simulink model "Day_07_LQR_with_Energy_Shaping"  (R2024a)
settings: Solver=daessc  StartTime=0.0  StopTime=5  RelTol=1e-3
values from neighbouring files (symbols this model uses):
  D0 = 2700    [Day_07.m]
  D1 = 2700    [Day_07.m]
  K = 20    [Day_07.m]
  K_LQR = lqr(A, B, Q, R)    [Day_07.m]
  L0 = 0.01    [Day_07.m]
  L1 = 0.14    [Day_07.m]
  limit = 0.45    [Day_07.m]
  M1 = L1*W1*T1*D1    (= 0.0378)    [Day_07.m]
  T0 = 0.01    [Day_07.m]
  T1 = 0.01    [Day_07.m]
  W0 = 0.01    [Day_07.m]
  W1 = 0.01    [Day_07.m]
  x1_d = 0    [Day_07.m]
  x2_d = 0    [Day_07.m]
  x3_d = 0    [Day_07.m]
  x4_d = 0    [Day_07.m]
undefined symbols (not defined in the file or in its folder): X, Y, Z
libraries: sm_lib x14, nesl_utility x7
settings Model: Creator=mingeun  LastModifiedBy=mingeun
settings DataIOCC: ReturnWorkspaceOutputs=off
settings OptimizationCC: BlockReduction=off  DefaultParameterBehavior=Inlined  BufferReuse=off

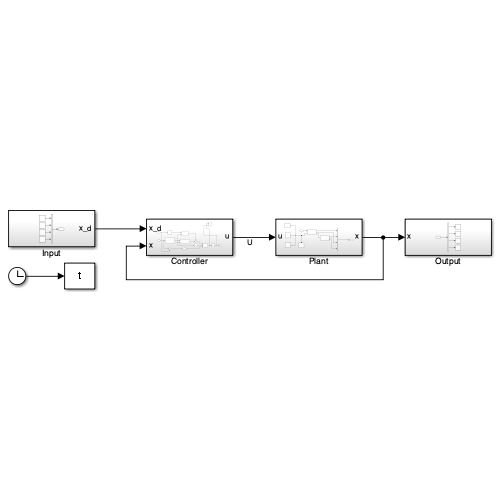
[thumbnail: Simulink's stored preview of the top-level diagram]
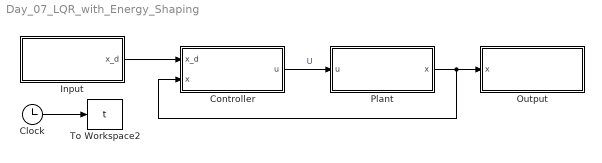
== system Day_07_LQR_with_Energy_Shaping ==
  Clock : Clock
  Controller : Subsystem
  Input : Subsystem
  Output : Subsystem
  Plant : Subsystem
  To Workspace2 : ToWorkspace  VariableName=t  SampleTime=-1
  wires:
  Clock/1 -> To Workspace2/1
  Input/1(x_d) -> Controller/1(x_d)
  Controller/1(u) -> Plant/1(u)  "U"
  Plant/1(x) -> Output/1(x), Controller/2(x)

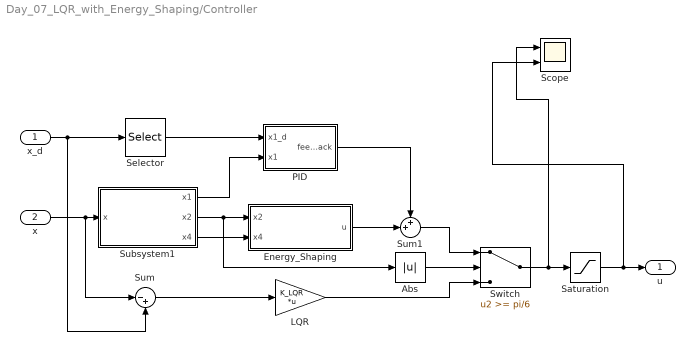
== system Day_07_LQR_with_Energy_Shaping/Controller ==
  x_d : Inport
  x : Inport  Port=2
  Abs : Abs  SaturateOnIntegerOverflow=off
  Energy_Shaping : Subsystem
  LQR : Gain  Gain=K_LQR  Multiplication=Matrix(K*u)
  PID : Subsystem  mask{Kp=2, Ki=0.02, Kd=0.2}
  Saturation : Saturate  UpperLimit=limit  LowerLimit=-limit
  Scope : Scope  NumInputPorts=2
  Selector : Selector  InputPortWidth=4  IndexOptions=Index vector (dialog)  Indices=1  OutputSizes=1
  Subsystem1 : Subsystem
  Sum : Sum  Inputs=|-+
  Sum1 : Sum  Inputs=++|
  Switch : Switch  Threshold=pi/6  SaturateOnIntegerOverflow=off  InputSameDT=off
  u : Outport
  wires:
  Switch/1 -> Scope/1, Saturation/1
  x_d/1 -> Sum/2, Selector/1
  Abs/1 -> Switch/2
  Sum1/1 -> Switch/1
  x/1 -> Subsystem1/1(x), Sum/1
  Subsystem1/3(x4) -> Energy_Shaping/2(x4)
  Energy_Shaping/1(u) -> Sum1/2
  Subsystem1/2(x2) -> Energy_Shaping/1(x2), Abs/1
  Subsystem1/1(x1) -> PID/2(x1)
  Sum/1 -> LQR/1
  Selector/1 -> PID/1(x1_d)
  PID/1(feedback) -> Sum1/1
  LQR/1 -> Switch/3
  Saturation/1 -> Scope/2, u/1

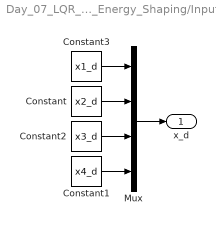
== system Day_07_LQR_with_Energy_Shaping/Input ==
  Constant : Constant  Value=x2_d
  Constant1 : Constant  Value=x4_d
  Constant2 : Constant  Value=x3_d
  Constant3 : Constant  Value=x1_d
  Mux : Mux
  x_d : Outport
  wires:
  Mux/1 -> x_d/1
  Constant1/1 -> Mux/4
  Constant2/1 -> Mux/3
  Constant/1 -> Mux/2
  Constant3/1 -> Mux/1

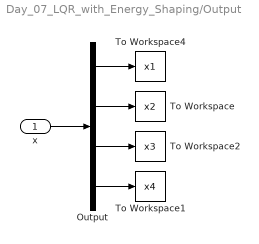
== system Day_07_LQR_with_Energy_Shaping/Output ==
  x : Inport
  Output : Demux
  To Workspace : ToWorkspace  VariableName=x2  SampleTime=-1
  To Workspace1 : ToWorkspace  VariableName=x4  SampleTime=-1
  To Workspace2 : ToWorkspace  VariableName=x3  SampleTime=-1
  To Workspace4 : ToWorkspace  VariableName=x1  SampleTime=-1
  wires:
  Output/3 -> To Workspace2/1
  Output/4 -> To Workspace1/1
  Output/2 -> To Workspace/1
  Output/1 -> To Workspace4/1
  x/1 -> Output/1

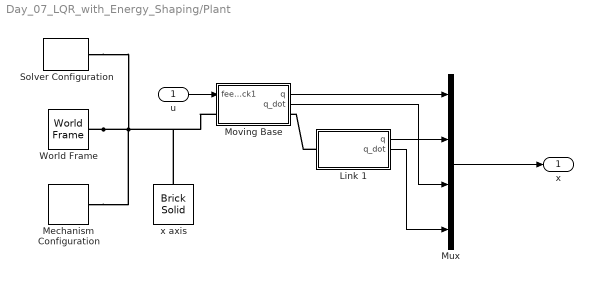
== system Day_07_LQR_with_Energy_Shaping/Plant ==
  u : Inport
  Link 1 : Subsystem  mask{L=L1*100, W=W1*100, H=T1*100, rho=D1, rgb=[0.25 0.40 0.70], angle=180, F=0.1}
      mask prompts: L "Length (cm)"; W "Width (cm)"; H "Thickness (cm)"; rho "Density (kg/m^3)"; rgb "Color [R G B]"; angle "Initial Angle (degree)"; F "Disturbance [N]"
  Mechanism Configuration : sm_lib/Utilities/Mechanism Configuration  UniformGravity=Constant  GravityVector=[0 0 -9.80665]  GravityVectorUnits=m/s^2  LinearizationDelta=0.001  JointModeTransitionNonlinearIterations=2
  Moving Base : Subsystem  mask{L=L0*100, W=W0*100, H=T0*100, rho=D0, RGB=[0.8 0.45 0.0]}
      mask prompts: L "Length (cm)"; W "Width (cm)"; H "Thickness (cm)"; rho "Density (kg/m^3)"; RGB "Color [R G B]"
  Mux : Mux
  Solver Configuration : nesl_utility/Solver Configuration  PhysicalDomain=network_engine_domain  SubClassName=solver  LeftPortType=input  RightPortType=generic  Tones=[]  Harmonics=[]  SimulateNoise=off  Profile=off  UseLocalSampling=off  EnableSwitchedLinearOptims=on  FrequencyDomain=off  UseCCode=off  RelTol=0.001  AbsTol=0.001  MinStep=1e-09  ToWorkspace=off  RevertToSquareIcSolve=off  NumHomotopyIterations=100  PhasorMode=off  PhasorModeNumHarmonics=1  ConsistencySolver=NEWTON_XTOL_AFTER_FTOL  IndexReductionMethod=DerivativeReplacement  DoDC=off  ResidualTolerance=1e-09  ConsistencyTolSource=GLOBAL  ConsistencyAbsTol=0.001  ConsistencyRelTol=0.001  ConsistencyTolFactor=0.001  UseLocalSolver=off  LocalSolverChoice=NE_BACKWARD_EULER_ADVANCER  ResolveIndetEquations=on  FunctionEvalNumThread=1  LocalSolverSampleTime=0.001  DoFixedCost=off  MaxNonlinIter=3  MaxModeIter=2  ComputeImpulses=off  ImpulseIterations=2  LinearAlgebra=auto  LinearAlgebraNumThread=0  EquationFormulation=NE_TIME_EF  DelaysMemoryBudget=1024  AutomaticFiltering=on  FilteringTimeConstant=0.001  PartitionStorageMethod=AS_NEEDED  PartitionMemoryBudget=1024  PartitionMethod=ROBUST  MultibodyUseLocalSolver=off  MultibodyLocalSolverChoice=ODE1  MultibodyLocalSolverSampleTime=0.001
  World Frame : sm_lib/Frames and Transforms/World Frame
  x axis : sm_lib/Body Elements/Brick Solid  BrickDimensions=[1000 1 1]  BrickDimensionsUnits=mm  ExportEntireGeometry=off  InertiaType=CalculateFromGeometry  BasedOnType=Density  Density=1000  DensityUnits=kg/m^3  Mass=1  MassUnits=kg  CenterOfMass=[0 0 0]  CenterOfMassUnits=m  MomentsOfInertia=[1 1 1]  MomentsOfInertiaUnits=kg*m^2  ProductsOfInertia=[0 0 0]  ProductsOfInertiaUnits=kg*m^2  GraphicType=FromGeometry  MarkerShape=Sphere  MarkerSize=10  GraphicVisPropType=SimpleVisualProperties  GraphicDiffuseColor=[0.0 0.0 0.0]  GraphicOpacity=1  GraphicSpecularColor=[0.5 0.5 0.5 1.0]  GraphicAmbientColor=[0.15 0.15 0.15 1.0]  GraphicEmissiveColor=[0.0 0.0 0.0 1.0]  GraphicShininess=75  DoExposeReferenceFrame=on  SerializedFrames=<Frames/>
  x : Outport
  wires:
  Moving Base/1(q) -> Mux/1
  Link 1/1(q) -> Mux/2
  u/1 -> Moving Base/1(feedback1)
  Link 1/2(q_dot) -> Mux/4
  Moving Base/2(q_dot) -> Mux/3
  Mux/1 -> x/1
  connections:
  World Frame/RConn1 -- Solver Configuration/RConn1 -- Moving Base/LConn1 -- x axis/RConn1 -- Mechanism Configuration/RConn1
  Link 1/LConn1 -- Moving Base/RConn1

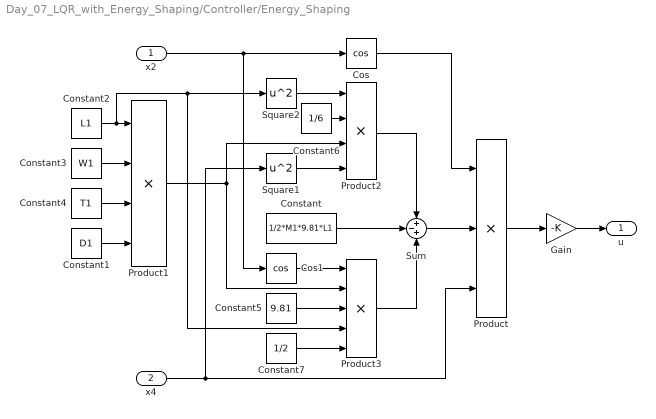
== system Day_07_LQR_with_Energy_Shaping/Controller/Energy_Shaping ==
  x2 : Inport
  x4 : Inport  Port=2
  Constant : Constant  Value=1/2*M1*9.81*L1
  Constant1 : Constant  Value=D1
  Constant2 : Constant  Value=L1
  Constant3 : Constant  Value=W1
  Constant4 : Constant  Value=T1
  Constant5 : Constant  Value=9.81
  Constant6 : Constant  Value=1/6
  Constant7 : Constant  Value=1/2
  Cos : Trigonometry  Operator=cos
  Cos1 : Trigonometry  Operator=cos
  Gain : Gain  Gain=-K
  Product : Product  Inputs=3
  Product1 : Product  Inputs=4
  Product2 : Product  Inputs=4
  Product3 : Product  Inputs=5
  Square1 : Math  Operator=square  SignedPower=on  RndMeth=Zero
  Square2 : Math  Operator=square  SignedPower=on  RndMeth=Zero
  Sum : Sum  Inputs=+-+
  u : Outport
  wires:
  Gain/1 -> u/1
  Sum/1 -> Product/2
  Cos/1 -> Product/1
  Product/1 -> Gain/1
  x4/1 -> Product/3, Square1/1
  x2/1 -> Cos1/1, Cos/1
  Constant2/1 -> Product3/4, Square2/1, Product1/1
  Constant3/1 -> Product1/2
  Constant4/1 -> Product1/3
  Constant1/1 -> Product1/4
  Product1/1 -> Product3/2, Product2/3
  Square1/1 -> Product2/4
  Product2/1 -> Sum/1
  Cos1/1 -> Product3/1
  Constant7/1 -> Product3/5
  Constant5/1 -> Product3/3
  Constant6/1 -> Product2/2
  Square2/1 -> Product2/1
  Constant/1 -> Sum/2
  Product3/1 -> Sum/3

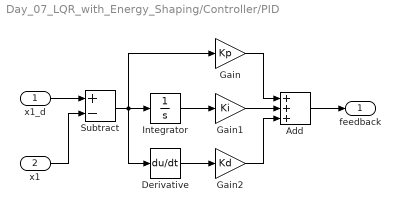
== system Day_07_LQR_with_Energy_Shaping/Controller/PID ==
  x1_d : Inport
  x1 : Inport  Port=2
  Add : Sum  Inputs=+++
  Derivative : Derivative
  Gain : Gain  Gain=Kp
  Gain1 : Gain  Gain=Ki
  Gain2 : Gain  Gain=Kd
  Integrator : Integrator
  Subtract : Sum  Inputs=+-
  feedback : Outport
  wires:
  x1_d/1 -> Subtract/1
  Derivative/1 -> Gain2/1
  Subtract/1 -> Integrator/1, Gain/1, Derivative/1
  Integrator/1 -> Gain1/1
  Add/1 -> feedback/1
  Gain/1 -> Add/1
  Gain2/1 -> Add/3
  Gain1/1 -> Add/2
  x1/1 -> Subtract/2

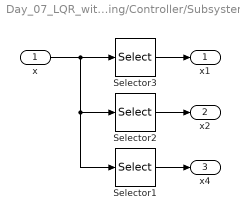
== system Day_07_LQR_with_Energy_Shaping/Controller/Subsystem1 ==
  x : Inport
  Selector1 : Selector  InputPortWidth=4  IndexOptions=Index vector (dialog)  Indices=4  OutputSizes=1
  Selector2 : Selector  InputPortWidth=4  IndexOptions=Index vector (dialog)  Indices=2  OutputSizes=1
  Selector3 : Selector  InputPortWidth=4  IndexOptions=Index vector (dialog)  Indices=1  OutputSizes=1
  x1 : Outport
  x2 : Outport  Port=2
  x4 : Outport  Port=3
  wires:
  Selector1/1 -> x4/1
  Selector2/1 -> x2/1
  Selector3/1 -> x1/1
  x/1 -> Selector2/1, Selector1/1, Selector3/1

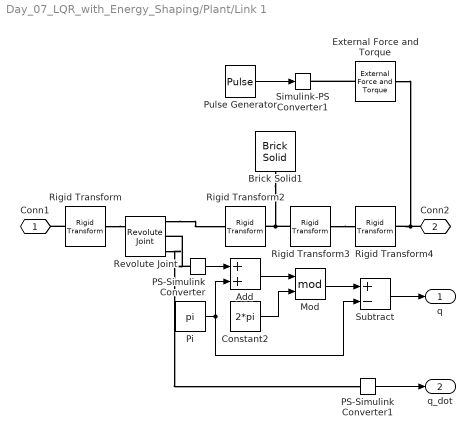
== system Day_07_LQR_with_Energy_Shaping/Plant/Link 1 ==
  Add : Sum
  Brick Solid1 : sm_lib/Body Elements/Brick Solid  BrickDimensions=[L W H]  BrickDimensionsUnits=cm  ExportEntireGeometry=off  InertiaType=CalculateFromGeometry  BasedOnType=Density  Density=rho  DensityUnits=kg/m^3  Mass=1  MassUnits=kg  CenterOfMass=[0 0 0]  CenterOfMassUnits=m  MomentsOfInertia=[1 1 1]  MomentsOfInertiaUnits=kg*m^2  ProductsOfInertia=[0 0 0]  ProductsOfInertiaUnits=kg*m^2  GraphicType=FromGeometry  MarkerShape=Sphere  MarkerSize=10  GraphicVisPropType=SimpleVisualProperties  GraphicDiffuseColor=rgb  GraphicOpacity=1  GraphicSpecularColor=[0.5 0.5 0.5 1.0]  GraphicAmbientColor=[0.15 0.15 0.15 1.0]  GraphicEmissiveColor=[0.0 0.0 0.0 1.0]  GraphicShininess=75  DoExposeReferenceFrame=on  SerializedFrames=<Frames/>
  Constant2 : Constant  Value=2*pi
  External Force and Torque : sm_lib/Forces and Torques/External Force and Torque  EnableForceX=on  EnableForceY=off  EnableForceZ=off  EnableForce=off  ForceResolutionFrame=World  EnableTorqueX=off  EnableTorqueY=off  EnableTorqueZ=off  EnableTorque=off  TorqueResolutionFrame=World
  Mod : Math  Operator=mod  OutputSignalType=real
  PS-Simulink Converter : nesl_utility/PS-Simulink Converter  PhysicalDomain=network_engine_domain  SubClassName=ps_output  LeftPortType=input  RightPortType=output  PseudoPeriodic=off  Frequencies=[]  VectorFormat=inherit  Unit=inherit  AffineConversion=off
  PS-Simulink Converter1 : nesl_utility/PS-Simulink Converter  PhysicalDomain=network_engine_domain  SubClassName=ps_output  LeftPortType=input  RightPortType=output  PseudoPeriodic=off  Frequencies=[]  VectorFormat=inherit  Unit=inherit  AffineConversion=off
  Pi : Constant  Value=pi  OutDataTypeStr=Inherit: Inherit via back propagation
  Pulse Generator : DiscretePulseGenerator  PulseType=Time based  Amplitude=F  Period=1000000  PulseWidth=1/1000000  PhaseDelay=0.25
  Revolute Joint : sm_lib/Joints/Revolute Joint  JointMode=Normal  CompositeWrenchDir=FollowerOnBase  CompositeWrenchFrame=BaseFrame  SenseConstraintForce=off  SenseConstraintTorque=off  SenseTotalForce=off  SenseTotalTorque=off  PositionTargetSpecify=on  PositionTargetPriority=High  PositionTargetValue=angle  PositionTargetValueUnits=deg  VelocityTargetSpecify=off  VelocityTargetPriority=High  VelocityTargetValue=0  VelocityTargetValueUnits=deg/s  EquilibriumPosition=0  EquilibriumPositionUnits=deg  SpringStiffness=0  SpringStiffnessUnits=N*m/deg  DampingCoefficient=0  DampingCoefficientUnits=N*m/(deg/s)  LowerLimitSpecify=off  LowerLimitBound=-90  LowerLimitBoundUnits=deg  LowerLimitStiffness=1e4  LowerLimitStiffnessUnits=N*m/deg  LowerLimitDamping=10  LowerLimitDampingUnits=N*m/(deg/s)  LowerLimitTransitionRegionWidth=0.1  LowerLimitTransitionRegionWidthUnits=deg  UpperLimitSpecify=off  UpperLimitBound=90  UpperLimitBoundUnits=deg  UpperLimitStiffness=1e4  UpperLimitStiffnessUnits=N*m/deg  UpperLimitDamping=10  UpperLimitDampingUnits=N*m/(deg/s)  UpperLimitTransitionRegionWidth=0.1  UpperLimitTransitionRegionWidthUnits=deg  TorqueActuationMode=InputTorque  MotionActuationMode=ComputedMotion  SensePosition=on  SenseVelocity=on  SenseAcceleration=off  SenseTorqueForce=off  SenseLowerLimitTorqueForce=off  SenseUpperLimitTorqueForce=off
  Rigid Transform : sm_lib/Frames and Transforms/Rigid Transform  RotationMethod=RotationMatrix  FollAlignAxisA=+X  BaseAlignAxisA=+Y  FollAlignAxisB=+Y  BaseAlignAxisB=+Z  RotationStandardAxis=+X  RotationAngle=90  RotationAngleUnits=deg  RotationArbitraryAxis=[0 0 1]  RotationSequenceAxes=FollowerAxes  RotationSequence=XYX  RotationSequenceAngles=[0 0 0]  RotationSequenceAnglesUnits=deg  RotationMatrix=[0 0 1; -1 0 0; 0 -1 0]  Quaternion=[1 0 0 0]  TranslationMethod=None  TranslationCartesianOffset=[0 0 0]  TranslationCartesianOffsetUnits=m  TranslationStandardAxis=+Z  TranslationStandardOffset=0  TranslationStandardOffsetUnits=m  TranslationROffset=0  TranslationROffsetUnits=m  TranslationThetaOffset=0  TranslationThetaOffsetUnits=deg  TranslationZOffset=0  TranslationZOffsetUnits=m
  Rigid Transform2 : sm_lib/Frames and Transforms/Rigid Transform  RotationMethod=None  FollAlignAxisA=+X  BaseAlignAxisA=+Y  FollAlignAxisB=+Y  BaseAlignAxisB=+Z  RotationStandardAxis=+Z  RotationAngle=0  RotationAngleUnits=deg  RotationArbitraryAxis=[0 0 1]  RotationSequenceAxes=FollowerAxes  RotationSequence=XYX  RotationSequenceAngles=[0 0 0]  RotationSequenceAnglesUnits=deg  RotationMatrix=[1 0 0;0 1 0;0 0 1]  Quaternion=[1 0 0 0]  TranslationMethod=StandardAxis  TranslationCartesianOffset=[0 0 0]  TranslationCartesianOffsetUnits=m  TranslationStandardAxis=-X  TranslationStandardOffset=L/2  TranslationStandardOffsetUnits=cm  TranslationROffset=0  TranslationROffsetUnits=m  TranslationThetaOffset=0  TranslationThetaOffsetUnits=deg  TranslationZOffset=0  TranslationZOffsetUnits=m
  Rigid Transform3 : sm_lib/Frames and Transforms/Rigid Transform  RotationMethod=None  FollAlignAxisA=+X  BaseAlignAxisA=+Y  FollAlignAxisB=+Y  BaseAlignAxisB=+Z  RotationStandardAxis=+Z  RotationAngle=0  RotationAngleUnits=deg  RotationArbitraryAxis=[0 0 1]  RotationSequenceAxes=FollowerAxes  RotationSequence=XYX  RotationSequenceAngles=[0 0 0]  RotationSequenceAnglesUnits=deg  RotationMatrix=[1 0 0;0 1 0;0 0 1]  Quaternion=[1 0 0 0]  TranslationMethod=StandardAxis  TranslationCartesianOffset=[0 0 0]  TranslationCartesianOffsetUnits=m  TranslationStandardAxis=-X  TranslationStandardOffset=L/2  TranslationStandardOffsetUnits=cm  TranslationROffset=0  TranslationROffsetUnits=m  TranslationThetaOffset=0  TranslationThetaOffsetUnits=deg  TranslationZOffset=0  TranslationZOffsetUnits=m
  Rigid Transform4 : sm_lib/Frames and Transforms/Rigid Transform  RotationMethod=None  FollAlignAxisA=+X  BaseAlignAxisA=+Y  FollAlignAxisB=+Y  BaseAlignAxisB=+Z  RotationStandardAxis=+Z  RotationAngle=0  RotationAngleUnits=deg  RotationArbitraryAxis=[0 0 1]  RotationSequenceAxes=FollowerAxes  RotationSequence=XYX  RotationSequenceAngles=[0 0 0]  RotationSequenceAnglesUnits=deg  RotationMatrix=[1 0 0; 0 0 1; 0 -1 0]  Quaternion=[1 0 0 0]  TranslationMethod=StandardAxis  TranslationCartesianOffset=[0 0 0]  TranslationCartesianOffsetUnits=m  TranslationStandardAxis=+X  TranslationStandardOffset=L  TranslationStandardOffsetUnits=cm  TranslationROffset=0  TranslationROffsetUnits=m  TranslationThetaOffset=0  TranslationThetaOffsetUnits=deg  TranslationZOffset=0  TranslationZOffsetUnits=m
  Simulink-PS Converter1 : nesl_utility/Simulink-PS Converter  PhysicalDomain=network_engine_domain  SubClassName=ps_input  LeftPortType=input  RightPortType=output  PseudoPeriodic=off  Frequencies=[]  NoiseDistribution=none  NoiseParameters=[]  Unit=1  AffineConversion=off  FilteringAndDerivatives=provide  SimscapeFilterOrder=1  InputFilterTimeConstant=0.001  UdotUserProvided=0
  Subtract : Sum  Inputs=+-
  Conn1 : PMIOPort  Side=Left
  Conn2 : PMIOPort  Port=2  Side=Right
  q : Outport
  q_dot : Outport  Port=2
  wires:
  Pulse Generator/1 -> Simulink-PS Converter1/1
  Mod/1 -> Subtract/1
  Constant2/1 -> Mod/2
  Pi/1 -> Subtract/2, Add/2
  PS-Simulink Converter/1 -> Add/1
  Add/1 -> Mod/1
  Subtract/1 -> q/1
  PS-Simulink Converter1/1 -> q_dot/1
  connections:
  PS-Simulink Converter/LConn1 -- Revolute Joint/RConn2
  Rigid Transform3/RConn1 -- Rigid Transform4/LConn1
  Rigid Transform/LConn1 -- Revolute Joint/LConn1
  Rigid Transform3/LConn1 -- Brick Solid1/RConn1 -- Rigid Transform2/LConn1
  Conn2/RConn1 -- External Force and Torque/RConn1 -- Rigid Transform4/RConn1
  Rigid Transform/RConn1 -- Conn1/RConn1
  Revolute Joint/RConn1 -- Rigid Transform2/RConn1
  External Force and Torque/LConn1 -- Simulink-PS Converter1/RConn1
  Revolute Joint/RConn3 -- PS-Simulink Converter1/LConn1

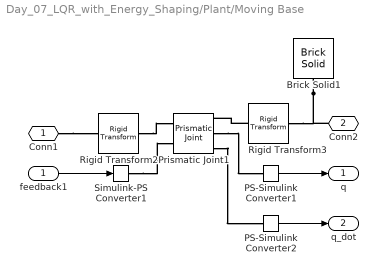
== system Day_07_LQR_with_Energy_Shaping/Plant/Moving Base ==
  feedback1 : Inport
  Brick Solid1 : sm_lib/Body Elements/Brick Solid  BrickDimensions=[L W H]  BrickDimensionsUnits=cm  ExportEntireGeometry=off  InertiaType=CalculateFromGeometry  BasedOnType=Density  Density=rho  DensityUnits=kg/m^3  Mass=1  MassUnits=kg  CenterOfMass=[0 0 0]  CenterOfMassUnits=m  MomentsOfInertia=[1 1 1]  MomentsOfInertiaUnits=kg*m^2  ProductsOfInertia=[0 0 0]  ProductsOfInertiaUnits=kg*m^2  GraphicType=FromGeometry  MarkerShape=Sphere  MarkerSize=10  GraphicVisPropType=SimpleVisualProperties  GraphicDiffuseColor=RGB  GraphicOpacity=1  GraphicSpecularColor=[0.5 0.5 0.5 1.0]  GraphicAmbientColor=[0.15 0.15 0.15 1.0]  GraphicEmissiveColor=[0.0 0.0 0.0 1.0]  GraphicShininess=75  DoExposeReferenceFrame=on  SerializedFrames=<Frames/>
  PS-Simulink Converter1 : nesl_utility/PS-Simulink Converter  PhysicalDomain=network_engine_domain  SubClassName=ps_output  LeftPortType=input  RightPortType=output  PseudoPeriodic=off  Frequencies=[]  VectorFormat=inherit  Unit=inherit  AffineConversion=off
  PS-Simulink Converter2 : nesl_utility/PS-Simulink Converter  PhysicalDomain=network_engine_domain  SubClassName=ps_output  LeftPortType=input  RightPortType=output  PseudoPeriodic=off  Frequencies=[]  VectorFormat=inherit  Unit=inherit  AffineConversion=off
  Prismatic Joint1 : sm_lib/Joints/Prismatic Joint  JointMode=Normal  CompositeWrenchDir=FollowerOnBase  CompositeWrenchFrame=BaseFrame  SenseConstraintForce=off  SenseConstraintTorque=off  SenseTotalForce=off  SenseTotalTorque=off  PositionTargetSpecify=off  PositionTargetPriority=High  PositionTargetValue=0  PositionTargetValueUnits=m  VelocityTargetSpecify=off  VelocityTargetPriority=High  VelocityTargetValue=0  VelocityTargetValueUnits=m/s  EquilibriumPosition=0  EquilibriumPositionUnits=m  SpringStiffness=0  SpringStiffnessUnits=N/m  DampingCoefficient=0  DampingCoefficientUnits=N/(m/s)  LowerLimitSpecify=off  LowerLimitBound=-1  LowerLimitBoundUnits=m  LowerLimitStiffness=1e6  LowerLimitStiffnessUnits=N/m  LowerLimitDamping=1e3  LowerLimitDampingUnits=N/(m/s)  LowerLimitTransitionRegionWidth=1e-4  LowerLimitTransitionRegionWidthUnits=m  UpperLimitSpecify=off  UpperLimitBound=1  UpperLimitBoundUnits=m  UpperLimitStiffness=1e6  UpperLimitStiffnessUnits=N/m  UpperLimitDamping=1e3  UpperLimitDampingUnits=N/(m/s)  UpperLimitTransitionRegionWidth=1e-4  UpperLimitTransitionRegionWidthUnits=m  TorqueActuationMode=InputTorque  MotionActuationMode=ComputedMotion  SensePosition=on  SenseVelocity=on  SenseAcceleration=off  SenseTorqueForce=off  SenseLowerLimitTorqueForce=off  SenseUpperLimitTorqueForce=off
  Rigid Transform2 : sm_lib/Frames and Transforms/Rigid Transform  RotationMethod=StandardAxis  FollAlignAxisA=+X  BaseAlignAxisA=+Y  FollAlignAxisB=+Y  BaseAlignAxisB=+Z  RotationStandardAxis=+Y  RotationAngle=90  RotationAngleUnits=deg  RotationArbitraryAxis=[0 0 1]  RotationSequenceAxes=FollowerAxes  RotationSequence=XYX  RotationSequenceAngles=[0 0 0]  RotationSequenceAnglesUnits=deg  RotationMatrix=[1 0 0;0 1 0;0 0 1]  Quaternion=[1 0 0 0]  TranslationMethod=None  TranslationCartesianOffset=[0 0 0]  TranslationCartesianOffsetUnits=m  TranslationStandardAxis=+Z  TranslationStandardOffset=0  TranslationStandardOffsetUnits=m  TranslationROffset=0  TranslationROffsetUnits=m  TranslationThetaOffset=0  TranslationThetaOffsetUnits=deg  TranslationZOffset=0  TranslationZOffsetUnits=m
  Rigid Transform3 : sm_lib/Frames and Transforms/Rigid Transform  RotationMethod=StandardAxis  FollAlignAxisA=+X  BaseAlignAxisA=+Y  FollAlignAxisB=+Y  BaseAlignAxisB=+Z  RotationStandardAxis=+Y  RotationAngle=90  RotationAngleUnits=deg  RotationArbitraryAxis=[0 0 1]  RotationSequenceAxes=FollowerAxes  RotationSequence=XYX  RotationSequenceAngles=[0 0 0]  RotationSequenceAnglesUnits=deg  RotationMatrix=[1 0 0;0 1 0;0 0 1]  Quaternion=[1 0 0 0]  TranslationMethod=None  TranslationCartesianOffset=[0 0 0]  TranslationCartesianOffsetUnits=m  TranslationStandardAxis=+Z  TranslationStandardOffset=0  TranslationStandardOffsetUnits=m  TranslationROffset=0  TranslationROffsetUnits=m  TranslationThetaOffset=0  TranslationThetaOffsetUnits=deg  TranslationZOffset=0  TranslationZOffsetUnits=m
  Simulink-PS Converter1 : nesl_utility/Simulink-PS Converter  PhysicalDomain=network_engine_domain  SubClassName=ps_input  LeftPortType=input  RightPortType=output  PseudoPeriodic=off  Frequencies=[]  NoiseDistribution=none  NoiseParameters=[]  Unit=1  AffineConversion=off  FilteringAndDerivatives=provide  SimscapeFilterOrder=1  InputFilterTimeConstant=0.001  UdotUserProvided=0
  Conn1 : PMIOPort  Side=Left
  Conn2 : PMIOPort  Port=2  Side=Right
  q : Outport
  q_dot : Outport  Port=2
  wires:
  feedback1/1 -> Simulink-PS Converter1/1
  PS-Simulink Converter1/1 -> q/1
  PS-Simulink Converter2/1 -> q_dot/1
  connections:
  Brick Solid1/RConn1 -- Conn2/RConn1 -- Rigid Transform3/LConn1
  Rigid Transform2/RConn1 -- Prismatic Joint1/LConn1
  Prismatic Joint1/RConn2 -- PS-Simulink Converter1/LConn1
  Simulink-PS Converter1/RConn1 -- Prismatic Joint1/LConn2
  Conn1/RConn1 -- Rigid Transform2/LConn1
  Rigid Transform3/RConn1 -- Prismatic Joint1/RConn1
  Prismatic Joint1/RConn3 -- PS-Simulink Converter2/LConn1
